simulink model "SimCodeGen_mfun_model"  (R2023b)
settings: Solver=VariableStepAuto  StartTime=0.0  StopTime=10.0  RelTol=1e-3
values from neighbouring files (symbols this model uses):
  params = [l2 l3]    [A3_1_init_VorKin.m]    (also in A3_2_init_InvKin.m; init_InvKin.m)
settings Model: Creator=Flo  LastModifiedBy=Flo

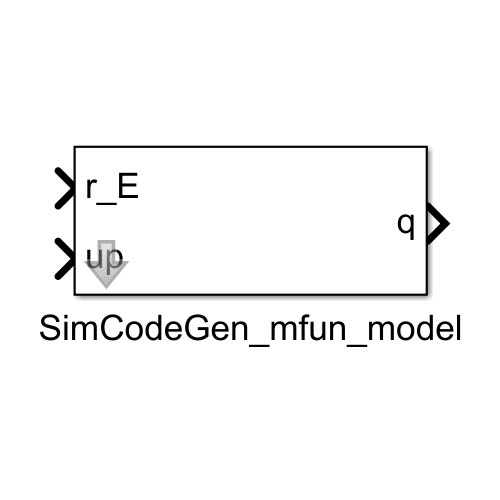
[thumbnail: Simulink's stored preview of the top-level diagram]
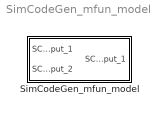
== system SimCodeGen_mfun_model ==
  SimCodeGen_mfun_model : Subsystem  mask{SC_param_0=params}
      mask prompts: SC_param_0 "params"
      mask Display:
      | port_label('input', 1, 'r_E');
      | port_label('input', 2, 'up');
      | port_label('output', 1, 'q');

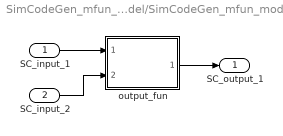
== system SimCodeGen_mfun_model/SimCodeGen_mfun_model ==
  SC_input_1 : Inport
  SC_input_2 : Inport  Port=2
  output_fun : MATLAB Function  TreatAsAtomicUnit=on
  SC_output_1 : Outport
  wires:
  output_fun/1(SC_output_0) -> SC_output_1/1
  SC_input_2/1 -> output_fun/2(SC_input_1)
  SC_input_1/1 -> output_fun/1(SC_input_0)

== matlab function SimCodeGen_mfun_model/output_fun ==
  data: SC_input_0 input size=[3]; SC_output_0 output size=[3]; SC_input_1 input size=[1]; SC_param_0 parameter size=[2]
function SC_output_0  = y_fun(SC_input_0, SC_input_1, SC_param_0)
    SC_output_0 = zeros(3,1);
    t1 = SC_input_0(3);
    t2 = SC_input_0(1);
    SC_output_0(1) = atan2(t1, t2);
    t4 = SC_input_0(2);
    t5 = t2 ^ 2;
    t6 = t1 ^ 2;
    t8 = sqrt(t5 + t6);
    t9 = atan2(t4, t8);
    t10 = SC_param_0(2);
    t11 = t4 ^ 2;
    t13 = sqrt(t5 + t11 + t6);
    t16 = SC_param_0(1);
    t17 = t16 ^ 2;
    t18 = t10 ^ 2;
    t19 = -t5 - t11 - t6 + t17 + t18;
    t20 = t19 ^ 2;
    t26 = sqrt(0.4e1 - 0.1e1 / t18 / t17 * t20);
    t29 = asin(t26 / t13 * t10 / 0.2e1);
    t31 = (-1) ^ SC_input_1(1);
    t32 = t31 * t29;
    SC_output_0(2) = pi / 0.2e1 - t9 + t32;
    t38 = acos(0.1e1 / t10 / t16 * t19 / 0.2e1);
    SC_output_0(3) = t9 - t32 + t31 * (pi - t38);
end
